simulink model "GliderResponseModel"  (R2013a)
settings: Solver=ode3  StartTime=0.0  StopTime=30  FixedStep=1e-2  RelTol=1e-3
libraries: simulink x5
settings Model: Creator=user  LastModifiedBy=user

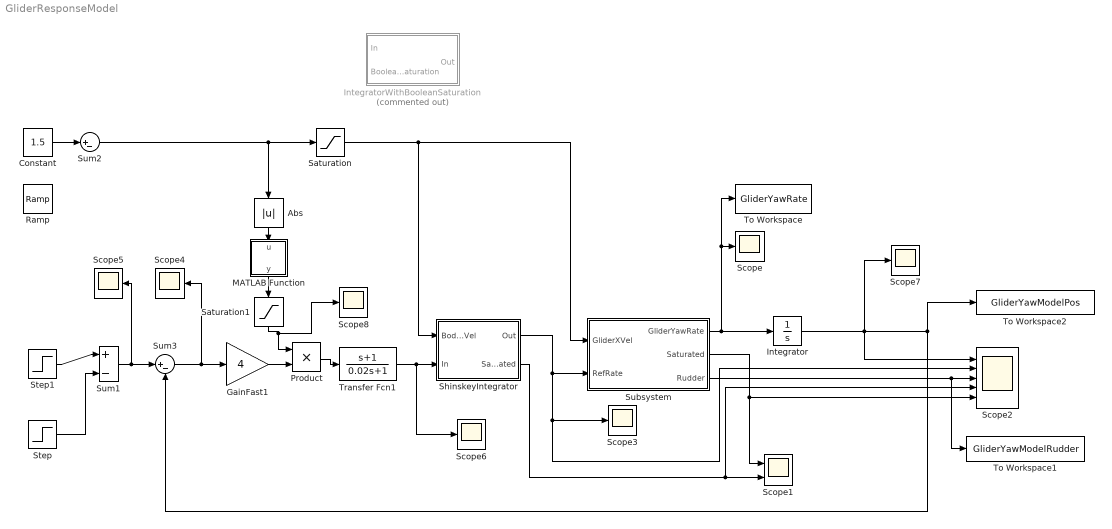
== system GliderResponseModel ==
  Abs : Abs
  Constant : Constant  Value=1.5
  GainFast1 : Gain  Gain=4
  Integrator : Integrator
  IntegratorWithBooleanSaturation : Subsystem  Commented=on
  MATLAB Function : MATLAB Function  TreatAsAtomicUnit=on
  Product : Product
  Ramp : simulink/Sources/Ramp  slope=0.005  start=5  X0=0
  Saturation : Saturate  UpperLimit=1.5  LowerLimit=0.1
  Saturation1 : Saturate  UpperLimit=1  LowerLimit=0.01
  Scope{,3..8} (7 alike) : Scope
      Scope settings: SaveName=ScopeData11
      Scope3 settings: YMin=-0.025  YMax=0.25  SaveName=ScopeData14
      Scope4 settings: SaveName=ScopeData16
      Scope5 settings: SaveName=ScopeData17
      Scope6 settings: YMin=-0.025  YMax=0.25  SaveName=ScopeData18
      Scope7 settings: SaveName=ScopeData19
      Scope8 settings: YMin=-0.025  YMax=0.25  SaveName=ScopeData21
  Scope1 : Scope  NumInputPorts=2
      settings: YMin=-5~-5  YMax=5~5  SaveName=ScopeData12
  Scope2 : Scope  NumInputPorts=5
      settings: ShowLegends=on  YMin=0.0986~-0.25~-0.75~-5~-5  YMax=0.0995~0.25~0.75~5~5  SaveName=ScopeData13
  ShinskeyIntegrator : Subsystem
  Step : Step  Time=7  After=0  SampleTime=0
  Step1 : Step  Time=5  After=0.1  SampleTime=0
  Subsystem : Subsystem
  Sum1 : Sum  Inputs=|+-
  Sum2 : Sum  Inputs=|+-
  Sum3 : Sum  Inputs=|+-
  To Workspace : ToWorkspace  VariableName=GliderYawRate  SampleTime=-1
  To Workspace1 : ToWorkspace  VariableName=GliderYawModelRudder  SampleTime=-1
  To Workspace2 : ToWorkspace  VariableName=GliderYawModelPos  SampleTime=-1
  Transfer Fcn1 : TransferFcn  Numerator=[1 1]  Denominator=[0.02 1]
  wires:
  Step1/1 -> Sum1/1
  Step/1 -> Sum1/2
  Constant/1 -> Sum2/1
  Sum2/1 -> Abs/1, Saturation/1
  Subsystem/1(GliderYawRate) -> Integrator/1, To Workspace/1, Scope/1
  Sum1/1 -> Scope5/1, Sum3/1
  Subsystem/2(Saturated) -> Scope2/5, Scope1/1
  Sum3/1 -> GainFast1/1, Scope4/1
  Transfer Fcn1/1 -> Scope6/1, ShinskeyIntegrator/2(In)
  GainFast1/1 -> Product/2
  ShinskeyIntegrator/1(Out) -> Scope2/2, Scope3/1, Subsystem/2(RefRate)
  ShinskeyIntegrator/2(Saturated) -> Scope2/4, Scope1/2
  Saturation/1 -> ShinskeyIntegrator/1(BodyFixedVel), Subsystem/1(GliderXVel)
  Subsystem/3(Rudder) -> To Workspace1/1, Scope2/3
  Integrator/1 -> Sum3/2, To Workspace2/1, Scope7/1, Scope2/1
  Saturation1/1 -> Scope8/1, Product/1
  Abs/1 -> MATLAB Function/1(u)
  MATLAB Function/1(y) -> Saturation1/1
  Product/1 -> Transfer Fcn1/1

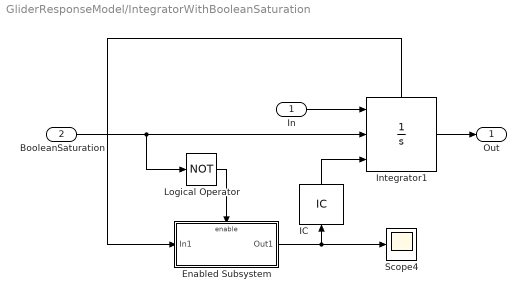
== system GliderResponseModel/IntegratorWithBooleanSaturation ==
  In : Inport
  BooleanSaturation : Inport  Port=2
  Enabled Subsystem : Subsystem  TreatAsAtomicUnit=on
  IC : InitialCondition  Value=0
  Integrator1 : Integrator  ExternalReset=level  InitialConditionSource=external  UpperSaturationLimit=5*pi/8  LowerSaturationLimit=-5*pi/8  ShowStatePort=on
  Logical Operator : Logic  Operator=NOT  AllPortsSameDT=off  OutDataTypeStr=boolean
  Scope4 : Scope
      settings: SaveName=ScopeData15
  Out : Outport
  wires:
  Enabled Subsystem/1(Out1) -> Scope4/1, IC/1
  In/1 -> Integrator1/1
  Integrator1/State -> Enabled Subsystem/1(In1)
  Integrator1/1 -> Out/1
  BooleanSaturation/1 -> Integrator1/2, Logical Operator/1
  Logical Operator/1 -> Enabled Subsystem/Enable
  IC/1 -> Integrator1/3

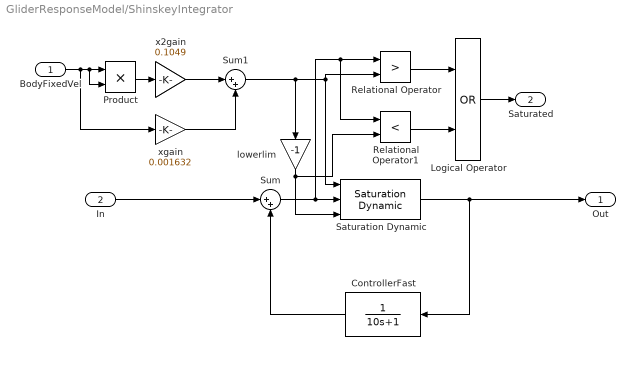
== system GliderResponseModel/ShinskeyIntegrator ==
  BodyFixedVel : Inport
  In : Inport  Port=2
  ControllerFast : TransferFcn  Denominator=[10 1]
  Logical Operator : Logic  Operator=OR  AllPortsSameDT=off  OutDataTypeStr=boolean
  Product : Product
  Relational Operator : RelationalOperator  Operator=>  OutDataTypeStr=boolean
  Relational Operator1 : RelationalOperator  Operator=<  OutDataTypeStr=boolean
  Saturation Dynamic : simulink/Discontinuities/Saturation Dynamic  OutMin=[]  OutMax=[]  OutDataTypeStr=Inherit: Same as second input  OutDataType=fixdt(1, 16)  OutScaling=2^-10  DoSatur=off
  Sum : Sum  Inputs=|++
  Sum1 : Sum  Inputs=|++
  lowerlim : Gain  Gain=-1
  x2gain : Gain  Gain=0.1049
  xgain : Gain  Gain=0.001632
  Out : Outport
  Saturated : Outport  Port=2
  wires:
  In/1 -> Sum/1
  Saturation Dynamic/1 -> ControllerFast/1, Out/1
  Sum/1 -> Relational Operator1/1, Relational Operator/1, Saturation Dynamic/2
  ControllerFast/1 -> Sum/2
  Sum1/1 -> lowerlim/1, Saturation Dynamic/1, Relational Operator/2
  lowerlim/1 -> Relational Operator1/2, Saturation Dynamic/3
  BodyFixedVel/1 -> xgain/1, Product/2, Product/1
  Product/1 -> x2gain/1
  x2gain/1 -> Sum1/1
  xgain/1 -> Sum1/2
  Relational Operator/1 -> Logical Operator/1
  Relational Operator1/1 -> Logical Operator/2
  Logical Operator/1 -> Saturated/1

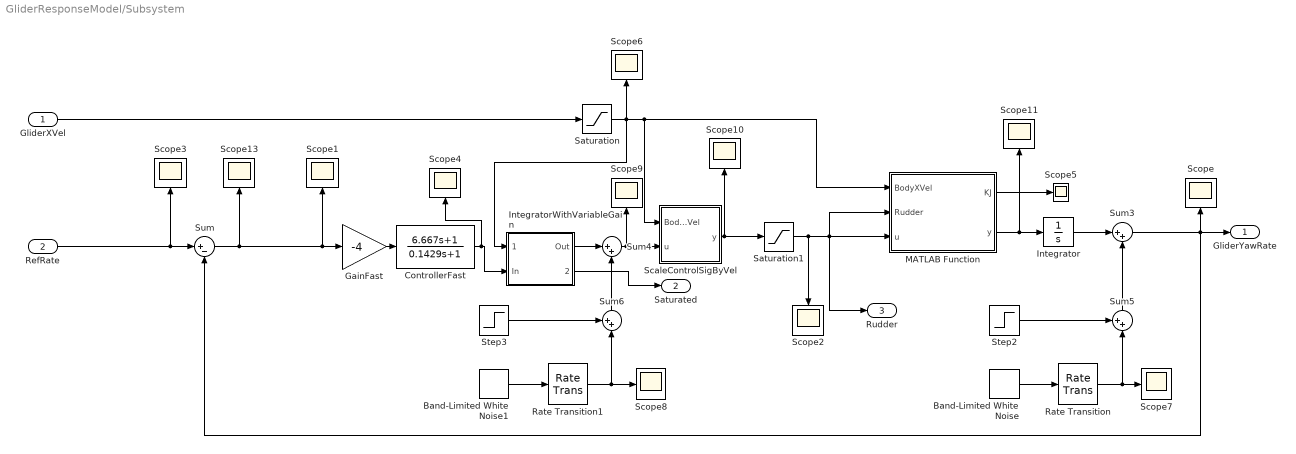
== system GliderResponseModel/Subsystem ==
  GliderXVel : Inport
  RefRate : Inport  Port=2
  Band-Limited White Noise : simulink/Sources/Band-Limited White Noise  Cov=[0.0000000]  Ts=0.01  seed=[23341]
  Band-Limited White Noise1 : simulink/Sources/Band-Limited White Noise  Cov=[0.000]  Ts=0.01  seed=[23341]
  ControllerFast : TransferFcn  Numerator=[6.667 1]  Denominator=[0.1429 1]
  GainFast : Gain  Gain=-4
  Integrator : Integrator
  IntegratorWithVariableGain : Subsystem
  MATLAB Function : MATLAB Function  TreatAsAtomicUnit=on
  Rate Transition : RateTransition
  Rate Transition1 : RateTransition
  Saturation : Saturate  UpperLimit=1.5  LowerLimit=0.1
  Saturation1 : Saturate  UpperLimit=pi/18*5  LowerLimit=-pi/18*5
  ScaleControlSigByVel : MATLAB Function  TreatAsAtomicUnit=on
  Scope{,1..11,13} (13 alike) : Scope
      Scope settings: TimeRange=60  YMin=0  YMax=0.225
      Scope10 settings: TimeRange=120  YMin=-1  YMax=0.4000000000000001  SaveName=ScopeData10
      Scope11 settings: TimeRange=60  YMin=0  YMax=0.225  SaveName=ScopeData20
      Scope13 settings: SaveName=ScopeData23
      Scope2 settings: TimeRange=120  YMin=-1  YMax=0.4000000000000001  SaveName=ScopeData2
      Scope3 settings: SaveName=ScopeData3
      Scope4 settings: YMax=1  SaveName=ScopeData4
      Scope5 settings: SaveName=ScopeData5
      Scope6 settings: SaveName=ScopeData6
      Scope7 settings: SaveName=ScopeData7
      Scope8 settings: YMin=-1.25  YMax=1.25  SaveName=ScopeData8
      Scope9 settings: SaveName=ScopeData9
  Step2 : Step  Time=40  After=0.00  SampleTime=0
  Step3 : Step  Time=80  After=0.0  SampleTime=0
  Sum : Sum  Inputs=|+-
  Sum3 : Sum  Inputs=|++
  Sum4 : Sum  Inputs=|++
  Sum5 : Sum  Inputs=++|
  Sum6 : Sum  Inputs=++|
  GliderYawRate : Outport
  Saturated : Outport  Port=2
  Rudder : Outport  Port=3
  wires:
  Step3/1 -> Sum6/1
  Band-Limited White Noise1/1 -> Rate Transition1/1
  IntegratorWithVariableGain/2(Saturated) -> Saturated/1
  ControllerFast/1 -> IntegratorWithVariableGain/2(In), Scope4/1
  MATLAB Function/1(KJ) -> Scope5/1
  Rate Transition1/1 -> Scope8/1, Sum6/2
  RefRate/1 -> Scope3/1, Sum/1
  MATLAB Function/2(y) -> Scope11/1, Integrator/1
  GliderXVel/1 -> Saturation/1
  Sum6/1 -> Sum4/2
  Rate Transition/1 -> Sum5/2, Scope7/1
  Integrator/1 -> Sum3/1
  GainFast/1 -> ControllerFast/1
  Band-Limited White Noise/1 -> Rate Transition/1
  Sum4/1 -> Scope9/1, ScaleControlSigByVel/2(u)
  Sum5/1 -> Sum3/2
  ScaleControlSigByVel/1(y) -> Saturation1/1, Scope10/1
  Step2/1 -> Sum5/1
  Saturation/1 -> IntegratorWithVariableGain/1(BodyXVel), ScaleControlSigByVel/1(BodyXVel), MATLAB Function/1(BodyXVel), Scope6/1
  IntegratorWithVariableGain/1(Out) -> Sum4/1
  Saturation1/1 -> MATLAB Function/2(Rudder), MATLAB Function/3(u), Rudder/1, Scope2/1
  Sum3/1 -> Scope/1, GliderYawRate/1, Sum/2
  Sum/1 -> Scope1/1, GainFast/1, Scope13/1

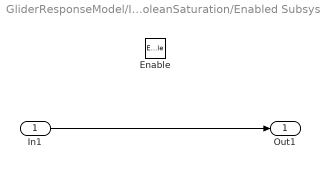
== system GliderResponseModel/IntegratorWithBooleanSaturation/Enabled Subsystem ==
  In1 : Inport
  Enable : EnablePort
  Out1 : Outport
  wires:
  In1/1 -> Out1/1

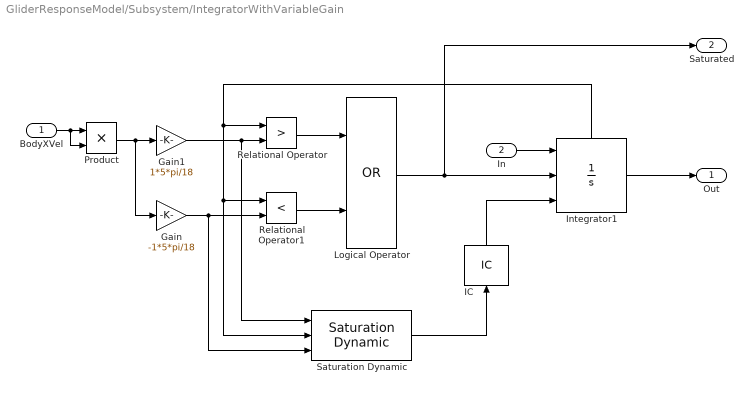
== system GliderResponseModel/Subsystem/IntegratorWithVariableGain ==
  BodyXVel : Inport
  In : Inport  Port=2
  Gain : Gain  Gain=-1*5*pi/18
  Gain1 : Gain  Gain=1*5*pi/18
  IC : InitialCondition  Value=0
  Integrator1 : Integrator  ExternalReset=level  InitialConditionSource=external  UpperSaturationLimit=5*pi/8  LowerSaturationLimit=-5*pi/8  ShowStatePort=on
  Logical Operator : Logic  Operator=OR  AllPortsSameDT=off  OutDataTypeStr=boolean
  Product : Product
  Relational Operator : RelationalOperator  Operator=>  OutDataTypeStr=boolean
  Relational Operator1 : RelationalOperator  Operator=<  OutDataTypeStr=boolean
  Saturation Dynamic : simulink/Discontinuities/Saturation Dynamic  OutMin=[]  OutMax=[]  OutDataTypeStr=Inherit: Same as second input  OutDataType=fixdt(1, 16)  OutScaling=2^-10  DoSatur=off
  Out : Outport
  Saturated : Outport  Port=2
  wires:
  In/1 -> Integrator1/1
  Integrator1/1 -> Out/1
  Relational Operator/1 -> Logical Operator/1
  Relational Operator1/1 -> Logical Operator/2
  Integrator1/State -> Relational Operator/1, Saturation Dynamic/2, Relational Operator1/1
  Gain1/1 -> Saturation Dynamic/1, Relational Operator/2
  Gain/1 -> Saturation Dynamic/3, Relational Operator1/2
  Logical Operator/1 -> Saturated/1, Integrator1/2
  Saturation Dynamic/1 -> IC/1
  IC/1 -> Integrator1/3
  BodyXVel/1 -> Product/2, Product/1
  Product/1 -> Gain/1, Gain1/1

== matlab function GliderResponseModel/MATLAB Function ==
  data: u input; y output
function y = fcn(u)
%#codegen

y = u;

== matlab function GliderResponseModel/Subsystem/MATLAB Function ==
  data: KJ output; BodyXVel input; Rudder input; u input; y output
function [KJ,y] = fcn(BodyXVel,Rudder,u)
%#codegen
RudderM = abs(Rudder);

% % First set of tests, long averaging time
% p00 =   0.0005488;
% p10 =    -0.03384;
% p01 =     0.02284;
% p20 =      0.1475;
% p11 =     -0.1365;
% p02 =    -0.02259;
% p30 =     -0.1176;
% p21 =     0.08015;
% p12 =    -0.04739;
% 
% 
% KJ = p00 + p10*RudderM + p01*BodyXVel + p20*RudderM^2 +...
%     p11*RudderM*BodyXVel + p02*BodyXVel^2 + p30*RudderM^3 +...
%     p21*RudderM^2*BodyXVel + p12*RudderM*BodyXVel^2;

% Second set of tests, short averaging time
p00 =    0.001019;
p10 =    -0.03252;
p01 =    0.007799;
p20 =      0.1448;
p11 =    -0.08634;
p02 =   -0.008142;
p30 =     -0.1309;
p21 =     0.09769;
p12 =     -0.1151;

KJ = p00 + p10*RudderM + p01*BodyXVel + p20*RudderM^2 + p11*RudderM*BodyXVel + p02*BodyXVel^2 ...
    + p30*RudderM^3 + p21*RudderM^2*BodyXVel + p12*RudderM*BodyXVel^2;

if KJ>-0.001
    KJ = -0.001;
end

y = KJ*u;

== matlab function GliderResponseModel/Subsystem/ScaleControlSigByVel ==
  data: BodyXVel input; u input; y output
function y = fcn(BodyXVel,u)
%#codegen

y = u/(BodyXVel^2);
